simulink model "battery_model"  (R2021a)
settings: Solver=VariableStepAuto  StartTime=0.0  StopTime=10.0  RelTol=1e-3
libraries: fl_lib x5, nesl_utility x5, ee_lib x1
settings Model: Creator=shubh  LastModifiedBy=LENOVO

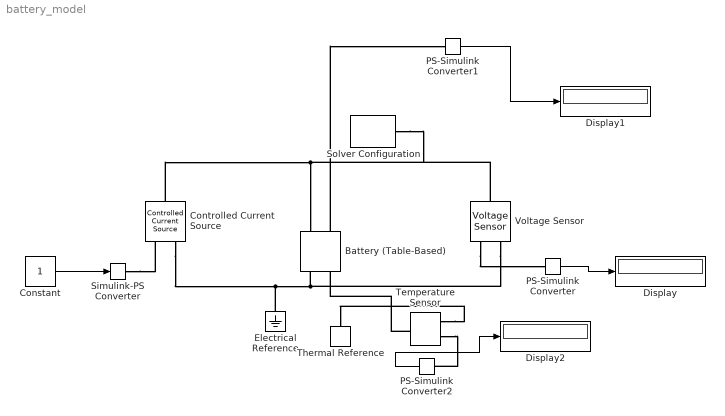
== system battery_model ==
  Battery (Table-Based) : ee_lib/Sources/Battery (Table-Based)  Tag={'toolbox/physmod/elec/library/m/ee_lib_parts';'Sources/Battery__Table_Based_/Panasonic/NCA103450.xml'}  SOC_vec=[0 0.01 0.02 0.03 0.04 0.05 0.06 0.07 0.08 0.09 0.1 0.11 0.12 0.13 0.14 0.15 0.16 0.17 0.18 0.19 0.2 0.21 0.22 0.23 0.24 0.25 0.26 0.27 0.28 0.29 0.3 0.31 0.32 0.33 0.34 0.35 0.36 0.37 0.38 0.39 0.4 0.41 0.42 0.43 0.44 0.45 0.46 0.47 0.48 0.49 0.5 0.51 0.52 0.53 0.54 0.55 0.56 0.57 0.58 0.59 0.6 0.61 0.62 0.63 0.64 0.65 0.66 0.67 0.68 0.69 0.7 0.71 0.72 0.73 0.74 0.75 0.76 0.77 0.78 0.79 0.8 0.81 0.82 0.83 0.84 0.85 0.86 0.87 0.88 0.89 0.9 0.91 0.92 0.93 0.94 0.95 0.96 0.97 0.98 0.99 1]  T_dependence=ee.enum.temperature_dependence.yes  prm_dir=ee.enum.battery.prm_dir.noCurrentDirectionality  T_vec=[-20 -10 0 25 40] degC  V0_mat=[3.05694324577171 3.05694324577171 3.05694324577171 3.05694324577171 3.05694324577171;3.11780933073521 3.11780933073521 3.11780933073521 3.11780933073521 3.11780933073521;3.16456091699536 3.16456091699536 3.16456091699536 3.16456091699536 3.16456091699536;3.20312763991407 3.20312763991407 3.20312763991407 3.20312763991407 3.20312763991407;3.23988086559703 3.23988086559703 3.23988086559703 3.23988086559703 3.23988086559703;3.27357083912107 3.27357083912107 3.27357083912107 3.27357083912107 3.27357083912107;3.29790581816648 3.29790581816648 3.29790581816648 3.29790581816648 3.29790581816648;3.31993534905873 3.31993534905873 3.31993534905873 3.31993534905873 3.31993534905873;3.34081960093889 3.34081960093889 3.34081960093889 3.34081960093889 3.34081960093889;3.35851365985912 3.35851365985912 3.35851365985912 3.35851365985912 3.35851365985912;3.37584043549754 3.37584043549754 3.37584043549754 3.37584043549754 3.37584043549754;3.39148360721865 3.39148360721865 3.39148360721865 3.39148360721865 3.39148360721865;3.40552818269083 3.40552818269083 3.40552818269083 3.40552818269083 3.40552818269083;3.41727372987041 3.41727372987041 3.41727372987041 3.41727372987041 3.41727372987041;3.42829270908039 3.42829270908039 3.42829270908039 3.42829270908039 3.42829270908039;3.43848498572673 3.43848498572673 3.43848498572673 3.43848498572673 3.43848498572673;3.44779771527731 3.44779771527731 3.44779771527731 3.44779771527731 3.44779771527731;3.45685827606495 3.45685827606495 3.45685827606495 3.45685827606495 3.45685827606495;3.46591883685259 3.46591883685259 3.46591883685259 3.46591883685259 3.46591883685259;3.47482240360815 3.47482240360815 3.47482240360815 3.47482240360815 3.47482240360815;3.48166780164756 3.48166780164756 3.48166780164756 3.48166780164756 3.48166780164756;3.48730800046594 3.48730800046594 3.48730800046594 3.48730800046594 3.48730800046594;3.49312425534464 3.49312425534464 3.49312425534464 3.49312425534464 3.49312425534464;3.49938346777656 3.49938346777656 3.49938346777656 3.49938346777656 3.49938346777656;3.50564268020849 3.50564268020849 3.50564268020849 3.50564268020849 3.50564268020849;3.51179877842532 3.51179877842532 3.51179877842532 3.51179877842532 3.51179877842532;3.5177347500538 3.5177347500538 3.5177347500538 3.5177347500538 3.5177347500538;3.52360520400279 3.52360520400279 3.52360520400279 3.52360520400279 3.52360520400279;3.5293131703325 3.5293131703325 3.5293131703325 3.5293131703325 3.5293131703325;3.53495846514988 3.53495846514988 3.53495846514988 3.53495846514988 3.53495846514988;3.54064002733928 3.54064002733928 3.54064002733928 3.54064002733928 3.54064002733928;3.5466862346196 3.5466862346196 3.5466862346196 3.5466862346196 3.5466862346196;3.55275206033938 3.55275206033938 3.55275206033938 3.55275206033938 3.55275206033938;3.55881788605916 3.55881788605916 3.55881788605916 3.55881788605916 3.55881788605916;3.56471104033438 3.56471104033438 3.56471104033438 3.56471104033438 3.56471104033438;3.57059107321653 3.57059107321653 3.57059107321653 3.57059107321653 3.57059107321653;3.57650036036778 3.57650036036778 3.57650036036778 3.57650036036778 3.57650036036778;3.58267113851687 3.58267113851687 3.58267113851687 3.58267113851687 3.58267113851687;3.58862363879637 3.58862363879637 3.58862363879637 3.58862363879637 3.58862363879637;3.59455112950322 3.59455112950322 3.59455112950322 3.59455112950322 3.59455112950322;3.60047862021008 3.60047862021008 3.60047862021008 3.60047862021008 3.60047862021008;3.60621921690956 3.60621921690956 3.60621921690956 3.60621921690956 3.60621921690956;3.61193277295345 3.61193277295345 3.61193277295345 3.61193277295345 3.61193277295345;3.61764632899735 3.61764632899735 3.61764632899735 3.61764632899735 3.61764632899735;3.62335988504124 3.62335988504124 3.62335988504124 3.62335988504124 3.62335988504124;3.62907344108513 3.62907344108513 3.62907344108513 3.62907344108513 3.62907344108513;3.63478699712903 3.63478699712903 3.63478699712903 3.63478699712903 3.63478699712903;3.64052178962629 ...(+4558 chars)] V  V0_vec=[3.05694324577171 3.11780933073521 3.16456091699536 3.20312763991407 3.23988086559703 3.27357083912107 3.29790581816648 3.31993534905873 3.34081960093889 3.35851365985912 3.37584043549754 3.39148360721865 3.40552818269083 3.41727372987041 3.42829270908039 3.43848498572673 3.44779771527731 3.45685827606495 3.46591883685259 3.47482240360815 3.48166780164756 3.48730800046594 3.49312425534464 3.49938346777656 3.50564268020849 3.51179877842532 3.5177347500538 3.52360520400279 3.5293131703325 3.53495846514988 3.54064002733928 3.5466862346196 3.55275206033938 3.55881788605916 3.56471104033438 3.57059107321653 3.57650036036778 3.58267113851687 3.58862363879637 3.59455112950322 3.60047862021008 3.60621921690956 3.61193277295345 3.61764632899735 3.62335988504124 3.62907344108513 3.63478699712903 3.64052178962629 3.64808511653063 3.65679215163517 3.66549918673971 3.6742776274848 3.68308819862471 3.69189876976462 3.70070934090453 3.70951991204444 3.71829251081983 3.72662762793713 3.73481883068441 3.74300361156379 3.75096334989971 3.75892308823563 3.76688282657154 3.77484256490746 3.78285738534165 3.79096087292362 3.79907208206368 3.80718329120375 3.81529450034382 3.82340570948388 3.83152467609174 3.83977969842631 3.84803472076089 3.85689864431254 3.8665947233018 3.87644566188505 3.88631890813263 3.89619215438021 3.90606540062778 3.91593864687536 3.92581189312294 3.93568513937051 3.94640464120662 3.95745251209717 3.96864585088705 3.98047153819836 3.9924662722967 4.00446100639504 4.01645574049338 4.02845047459172 4.03962340380677 4.05026614066205 4.06069004513023 4.07111394959842 4.08126368305597 4.09164730401325 4.10347838409614 4.11623674377326 4.12666159839296 4.13378671073504 4.05293761327992] V  R0_mat=[0.141685622669533 0.144330670296816 0.145951810032112 0.0876729363384268 0.146321047773631;0.160963346658006 0.160698886191678 0.150906802623426 0.0932229543109529 0.12440875553873;0.173825389417679 0.17065142085774 0.14944611398594 0.0950081088191402 0.108002561492024;0.182967039749425 0.176883563095875 0.144265032920527 0.0963551224210397 0.109029380824381;0.191284373155831 0.182291388408669 0.147971901771216 0.0982529232972309 0.109231883231397;0.198209319217276 0.188395970195294 0.152775341587345 0.100527086809133 0.108041998293454;0.202056790677236 0.190736653273694 0.153326511185911 0.100635443372933 0.102599843137946;0.205007765369114 0.192029405373389 0.152829749805771 0.100924551895045 0.105416708079588;0.207438158691858 0.19280157610395 0.151812407056497 0.101472051142568 0.108218448748171;0.208418464305548 0.192123659125456 0.152607874905011 0.101627556367249 0.109570101707698;0.209231822972955 0.19127879520068 0.153587839714389 0.101741529793572 0.110754807720943;0.210343575742801 0.191833133998348 0.153802530015898 0.101999894636474 0.111174239226319;0.210906938107855 0.191939665053811 0.153290585658805 0.101899166770183 0.110867036073093;0.210425287612639 0.191001183249004 0.151733628441442 0.101204214783437 0.109514820059597;0.209613378949417 0.18973244327619 0.149846413056072 0.101035811125123 0.107832345878095;0.208425696393633 0.188087929410814 0.147583423778142 0.100938308201256 0.105774097804031;0.206838219703417 0.186043621411006 0.144920640365778 0.100646635129898 0.1048982342853;0.205136120848225 0.183884691246222 0.144265334326882 0.100298317383989 0.104783849816211;0.204781000088455 0.18172576108144 0.144096514624598 0.0999499996380807 0.104669465347122;0.204845388629513 0.180789899114949 0.143856333998639 0.099556199105654 0.104483719954358;0.203974245935958 0.179205361561599 0.142680622138068 0.098627385343966 0.103362443326983;0.202555285414659 0.177073006180505 0.140957092449753 0.0976208329780398 0.101693348871863;0.201216350375327 0.175020676281377 0.139313588243404 0.0967773657175446 0.10010427989871;0.200078759678369 0.173169690724624 0.137871428379431 0.0963442210505122 0.0987165552679319;0.198941168981411 0.171318705167871 0.136429268515457 0.0959110763834798 0.0973288306371532;0.197756708186686 0.169420849513351 0.134940238553716 0.0954547691681331 0.0958942359086076;0.196472189851799 0.167422936318669 0.133351151051812 0.0949490149125893 0.0943595836398997;0.195157890753505 0.16539524236058 0.131732282786502 0.0944242795111379 0.0927951506077853;0.194078713655907 0.163293690393728 0.130039556512429 0.0939040760935132 0.0911568595669077;0.193117191689189 0.16189590605745 0.129087926592782 0.0933892475911817 0.0899127547919209;0.192172154891564 0.16081228938684 0.128373215654712 0.0929080144571439 0.0892588989120233;0.191392865862544 0.159894420484837 0.127824252485248 0.0927344186869696 0.0887707908007316;0.190622494306004 0.158985469055313 0.127284206788263 0.0925652298072645 0.0882916001619189;0.189852122749463 0.158076517625787 0.126744161091277 0.092396040927559 0.0878124095231052;0.189003264172671 0.157089079176012 0.126125628374041 0.0921768273536275 0.0872547318640409;0.188148441326298 0.156095676456655 0.125501131387224 0.0919538123771066 0.0866910899353958;0.187306915874968 0.155115571132341 0.12488993179545 0.091728288458123 0.0861407454017938;0.186584249968117 0.154254325352506 0.124397591748154 0.0914803382099938 0.0857092604126705;0.185973999931887 0.153293862359217 0.123806034487405 0.0911833561994023 0.0851785582100926;0.185407583884335 0.152322031378363 0.123203109239091 0.0908807562879789 0.0846364880199505;0.184841167836782 0.151350200397509 0.122600183990775 0.0905781563765555 0.0840944178298075;0.184189799967698 0.150293417595122 0.121806624470283 0.0901024318999258 0.0834673958181323;0.183526140891528 0.149405957488493 0.12081808813039 0.0896016589917948 0.0828280825993722;0.182862481815358 0.148580232764828 0.119829551790498 0.0891008860836628 0.0821887693806117 ...(+5198 chars)] Ohm  R0_vec=[0.0876729363384268 0.0932229543109529 0.0950081088191402 0.0963551224210397 0.0982529232972309 0.100527086809133 0.100635443372933 0.100924551895045 0.101472051142568 0.101627556367249 0.101741529793572 0.101999894636474 0.101899166770183 0.101204214783437 0.101035811125123 0.100938308201256 0.100646635129898 0.100298317383989 0.0999499996380807 0.099556199105654 0.098627385343966 0.0976208329780398 0.0967773657175446 0.0963442210505122 0.0959110763834798 0.0954547691681331 0.0949490149125893 0.0944242795111379 0.0939040760935132 0.0933892475911817 0.0929080144571439 0.0927344186869696 0.0925652298072645 0.092396040927559 0.0921768273536275 0.0919538123771066 0.091728288458123 0.0914803382099938 0.0911833561994023 0.0908807562879789 0.0905781563765555 0.0901024318999258 0.0896016589917948 0.0891008860836628 0.0886001131755307 0.0880993402673991 0.087598567359268 0.0871039468701925 0.0871146616224242 0.0872948764839462 0.0874750913454692 0.087721451026969 0.0879975738919554 0.0882736967569409 0.0885498196219272 0.0888259424869137 0.0890668906066512 0.0889393184390105 0.0888240888416965 0.0887072256611772 0.0885368621772216 0.0883664986932668 0.0881961352093101 0.0880257717253553 0.0879064321583712 0.0878659140766787 0.0878247337687346 0.0877835534607895 0.0877423731528449 0.0877011928449002 0.087661755097109 0.087652879550087 0.0876440040030652 0.0879694121511781 0.088545618141283 0.0891085428626062 0.0896695544051722 0.0902305659477382 0.0907915774903036 0.091352589032869 0.0919136005754355 0.092474612118 0.0932257180713086 0.0940612343386086 0.094932150401911 0.0962822749828668 0.0977889918051445 0.0992957086274227 0.100802425449702 0.10230914227198 0.10363125704595 0.104982100658977 0.106351712058201 0.107721323457427 0.108820835674904 0.109987805318691 0.111479917736467 0.112737722386497 0.109961816871439 0.104129278053125 0.01680404166307] Ohm  R0_dis_mat=[0.03 0.015 0.002;0.04 0.017 0.008;0.039 0.012 0.006;0.027 0.013 0.021] % Parameter not set Ohm  R0_dis_vec=[0.015 0.017 0.012 0.013] % Parameter not set Ohm  R0_ch_mat=[0.03 0.015 0.002;0.04 0.017 0.008;0.039 0.012 0.006;0.027 0.013 0.021] % Parameter not set Ohm  R0_ch_vec=[0.015 0.017 0.012 0.013] % Parameter not set Ohm  AH_vec=[1.55869476118114 1.8607446859296 2.01137468341514 2.193305986659 2.31762046623156] hr*A  AH=2.193305986659 hr*A  prm_leak=ee.enum.battery.prm_leak.disabled  Rleak_vec=[8000 7000 6000] % Parameter not set Ohm  Rleak=7000 % Parameter not set Ohm  extrapolation_option=ee.enum.extrapolation.nearest  prm_dyn=ee.enum.battery.prm_dyn.off  R1_mat=[0.089 0.076 0.01;0.042 0.022 0.099;0.019 0.007 0.002;0.051 0.043 0.029] % Parameter not set Ohm  R1_vec=[0.076 0.022 0.007 0.043] % Parameter not set Ohm  tau1_mat=[44 148 235;93 110 1000;19 27 133;0.5 22 3] % Parameter not set s  tau1_vec=[148 110 27 22] % Parameter not set s  R2_mat=[0.014 0.382 0.407;0.028 0.006 0.007;0.014 0.007 0.006;0.333 0.956 0.912] % Parameter not set Ohm  R2_vec=[0.382 0.006 0.007 0.956] % Parameter not set Ohm  tau2_mat=[1 44 5644;11 24 506;2 14 330;3310 13419 30216] % Parameter not set s  tau2_vec=[44 24 14 13419] % Parameter not set s  R3_mat=[0.014 0.382 0.407;0.028 0.006 0.007;0.014 0.007 0.006;0.333 0.956 0.912] % Parameter not set Ohm  R3_vec=[0.382 0.006 0.007 0.956] % Parameter not set Ohm  tau3_mat=[1 44 5644;11 24 506;2 14 330;3310 13419 30216] % Parameter not set s  tau3_vec=[44 24 14 13419] % Parameter not set s  R4_mat=[0.014 0.382 0.407;0.028 0.006 0.007;0.014 0.007 0.006;0.333 0.956 0.912] % Parameter not set Ohm  R4_vec=[0.382 0.006 0.007 0.956] % Parameter not set Ohm  tau4_mat=[1 44 5644;11 24 506;2 14 330;3310 13419 30216] % Parameter not set s  tau4_vec=[44 24 14 13419] % Parameter not set s  R5_mat=[0.014 0.382 0.407;0.028 0.006 0.007;0.014 0.007 0.006;0.333 0.956 0.912] % Parameter not set Ohm  R5_vec=[0.382 0.006 0.007 0.956] % Parameter not set Ohm  tau5_mat=[1 44 5644;11 24 506;2 14 330;3310 13419 30216] % Parameter not set s  tau5_vec=[44 24 14 13419] % Parameter not set s  prm_fade=ee.enum.battery.prm_fade.tableN  N0=100 % Parameter not set  dV0=0 % Parameter not set  dR0=0 % Parameter not set  dAH=0 % Parameter not set  dRleak=0 % Parameter not set  dR1=0 % Parameter not set  dR2=0 % Parameter not set  dR3=0 % Parameter not set  dR4=0 % Parameter not set  dR5=0 % Parameter not set  N0vec=[1 6 11 16 21 26 31 36 41 46 51 56 61 66 71 76 81 86 91 96 101 106 111 116 121 126 131 136 141 146 151 156 161 166 171 176 181 186 191 196 201 206 211 216 221 226 231 236 241 246 251 256 261 266 271 276 281 286 291 296 301 306 311 316 321 326 331 336 341 346 351 356 361 366 371 376 381 386 391 396 401 406 411 416 421 426 431 436 441 446 451 456 461 466 471 476 481 486 491 496]  Tfadevec=[298.15 323.15] % Parameter not set K  dV0vec=[0 1.10576459758607 1.97572945152668 1.87828003984863 1.76314184449295 1.62056220493866 1.56247815839591 1.52003609404217 1.47744416806089 1.43485224207961 1.39226031609831 1.34966839011701 1.30707646413573 1.26448453815445 1.22371856658483 1.18422222850361 1.14135385798404 1.09050719258034 1.0396605271766 0.988813861772903 0.940063540749295 0.895437648878542 0.85081175700779 0.806185865137015 0.761559973266241 0.71693408139551 0.672907210282603 0.629286501316299 0.585665792349996 0.542045083383692 0.506686498509871 0.471972266399757 0.436955084942783 0.4013031300697 0.365651175196617 0.329999220323534 0.294347265450451 0.258695310577368 0.223043355704285 0.187391400831202 0.151739445958163 0.11608749108508 0.0804355362120185 0.0447835813389573 0.00913162646587428 -0.0168261289375092 -0.035088995065174 -0.0533518611928607 -0.0717343945200007 -0.0903806588841135 -0.109026923248226 -0.127673187612339 -0.146319451976452 -0.164965716340565 -0.183611980704678 -0.202258245068791 -0.220904509432904 -0.239550773797016 -0.258197038161129 -0.279035070103965 -0.312374631634333 -0.346571377380647 -0.381571825677453 -0.41657227397426 -0.451572722271067 -0.486573170567873 -0.521573618864702 -0.556574067161487 -0.591574515458315 -0.628222003502564 -0.665796847356149 -0.703371691209755 -0.740946535063362 -0.776248754132794 -0.803500841123046 -0.830752928113297 -0.858005015103527 -0.885257102093779 -0.912509189084031 -0.939761276074282 -0.967013363064534 -0.994265450054808 -1.02151753704506 -1.04876962403531 -1.07602171102556 -1.10327379801584 -1.1303726689468 -1.14505002807567 -1.15972738720453 -1.17440474633339 -1.18908210546226 -1.20375946459112 -1.21843682371996 -1.23311418284882 -1.24779154197769 -1.26246890110655 -1.27714626023541 -1.29182361936425 -1.30650097849312 -1.32117833762196]  dR0vec=[0;0;0;0;0;0;0;0;0;0;0;0;0;0;0;0;0;0;0;0;0;0;0;0;0;0;0;0;0;0;0;0;0;0;0;0;0;0;0;0;0;0;0;0;0;0;0;0;0;0;0;0;0;0;0;0;0;0;0;0;0;0;0;0;0;0;0;0;0;0;0;0;0;0;0;0;0;0;0;0;0;0;0;0;0;0;0;0;0;0;0;0;0;0;0;0;0;0;0;0] % Parameter not set  dAHvec=[0 -0.554316012182733 -1.1086320243655 -1.66294803654826 -2.21726404873103 -2.77158006091378 -2.99739713515845 -3.13269855571741 -3.26799997627637 -3.40330139683531 -3.53860281739426 -3.67390423795322 -3.80920565851216 -3.94450707907112 -4.07980849963007 -4.21510992018901 -4.36196281111826 -4.53614670750021 -4.71033060388216 -4.88451450026413 -5.05869839664608 -5.23288229302803 -5.40706618940998 -5.58125008579193 -5.7554339821739 -5.92961787855585 -6.1038017749378 -6.27798567131975 -6.4521695677017 -6.62635346408365 -6.76754548571347 -6.90616451213779 -7.04478353856213 -7.18340256498647 -7.32202159141079 -7.46064061783513 -7.59925964425945 -7.73787867068379 -7.87649769710813 -8.01511672353245 -8.15373574995677 -8.29235477638112 -8.43097380280546 -8.56959282922977 -8.70821185565412 -8.80913868547283 -8.88014687370122 -8.95115506192963 -9.02216325015801 -9.0931714383864 -9.16417962661481 -9.23518781484319 -9.30619600307157 -9.37720419129998 -9.44821237952837 -9.51922056775675 -9.59022875598516 -9.66123694421355 -9.73224513244195 -9.81159994934316 -9.93856274544924 -10.0655255415553 -10.1924883376614 -10.3194511337675 -10.4464139298736 -10.5733767259797 -10.7003395220858 -10.8273023181919 -10.954265114298 -11.0812279104041 -11.2081907065101 -11.3351535026162 -11.4621162987223 -11.5814000530147 -11.6734829683154 -11.7655658836161 -11.8576487989168 -11.9497317142175 -12.0418146295181 -12.1338975448188 -12.2259804601195 -12.3180633754202 -12.4101462907209 -12.5022292060216 -12.5943121213223 -12.686395036623 -12.7779602454664 -12.8275540258614 -12.8771478062564 -12.9267415866515 -12.9763353670465 -13.0259291474415 -13.0755229278365 -13.1251167082315 -13.1747104886265 -13.2243042690216 -13.2738980494166 -13.3234918298116 -13.3730856102066 -13.4226793906016]  dRleakvec=[0 0 0] % Parameter not set  dR1vec=[0 0 0] % Parameter not set  dR2vec=[0 0 0] % Parameter not set  dR3vec=[0 0 0] % Parameter not set  dR4vec=[0 0 0] % Parameter not set  dR5vec=[0 0 0] % Parameter not set  dV0mat=[0 0;0 0;0 0] % Parameter not set  dR0mat=[0 0;0 0;0 0] % Parameter not set  dAHmat=[0 0;0 0;0 0] % Parameter not set  dRleakmat=[0 0;0 0;0 0] % Parameter not set  dR1mat=[0 0;0 0;0 0] % Parameter not set  dR2mat=[0 0;0 0;0 0] % Parameter not set  dR3mat=[0 0;0 0;0 0] % Parameter not set  dR4mat=[0 0;0 0;0 0] % Parameter not set  dR5mat=[0 0;0 0;0 0] % Parameter not set  prm_age=ee.enum.battery.prm_age.disabled  prm_age_OCV=ee.enum.battery.prm_age_OCV.SOC  OCV_age=0.9 % Parameter not set  SOC_age=0.6 % Parameter not set  storage_dt_age_vec=0 % Parameter not set d  storage_T_age_vec=273 % Parameter not set K  OCV_scaling_age=2213400 % Parameter not set  OCV_offset_age=1632000 % Parameter not set  temp_exp_age=0.515833569 % Parameter not set V  t_exp_age=0.75 % Parameter not set  T_age_vec=[273.15 298.15 323.15] % Parameter not set K  dt_age_vec=[90 180 270 360] % Parameter not set d  dR0_age_vec=[0 0 0] % Parameter not set  t_meas_dR0_age=100 % Parameter not set d  dR0_age_mat=[0 0 0;0 0 0;0 0 0;0 0 0] % Parameter not set  temperature=298.15 K  i_specify=off  i_priority=None  i=0 A  i_nominal_specify=off  i_nominal_unit=A  i_nominal_value=1  v_specify=off  v_priority=None  v=0 V  v_nominal_specify=off  v_nominal_unit=V  v_nominal_value=1  stateOfCharge_specify=off  stateOfCharge_priority=High  stateOfCharge=1  stateOfCharge_nominal_specify=off  stateOfCharge_nominal_unit=1  stateOfCharge_nominal_value=1  num_cycles_specify=off  num_cycles_priority=High  num_cycles=0  num_cycles_nominal_specify=off  num_cycles_nominal_unit=1  num_cycles_nominal_value=1  thermal_mass=30000 % Parameter not set J/K  temperature_specify=off  temperature_priority=High  temperature_nominal_specify=off  temperature_nominal_unit=K  temperature_nominal_value=1
      settings: AttributesFormatString=Panasonic:NCA103450  SourceProductBaseCode=PS  InternalSimscapePortConfiguration="{\"Bottom\":[],\"Left\":[{\"id\":\"p\",\"label\":\"+\",\"type\":\"foundation.electrical.electrical\"},{\"id\":\"soc\",\"label\":\"SOC\",\"type\":\"output\"}],\"Right\":[{\"id\":\"n\",\"label\":\"-\",\"type\":\"foundation.electrical.electrical\"},{\"id\":\"H\",\"label\":\"H\",\"type\":\"foundation.thermal.thermal\"}],\"Top\":[]}"
  Constant : Constant
  Controlled Current Source : fl_lib/Electrical/Electrical Sources/Controlled Current Source
  Display : Display
  Display1 : Display
  Display2 : Display
  Electrical Reference : fl_lib/Electrical/Electrical Elements/Electrical Reference
  PS-Simulink Converter : nesl_utility/PS-Simulink Converter  PhysicalDomain=network_engine_domain  SubClassName=ps_output  LeftPortType=input  RightPortType=output  PseudoPeriodic=off  Frequencies=[]  Unit=inherit  AffineConversion=off
      settings: SourceProductBaseCode=PW,SS
  PS-Simulink Converter1 : nesl_utility/PS-Simulink Converter  PhysicalDomain=network_engine_domain  SubClassName=ps_output  LeftPortType=input  RightPortType=output  PseudoPeriodic=off  Frequencies=[]  Unit=inherit  AffineConversion=off
      settings: SourceProductBaseCode=PW,SS
  PS-Simulink Converter2 : nesl_utility/PS-Simulink Converter  PhysicalDomain=network_engine_domain  SubClassName=ps_output  LeftPortType=input  RightPortType=output  PseudoPeriodic=off  Frequencies=[]  Unit=inherit  AffineConversion=off
      settings: SourceProductBaseCode=PW,SS
  Simulink-PS Converter : nesl_utility/Simulink-PS Converter  PhysicalDomain=network_engine_domain  SubClassName=ps_input  LeftPortType=input  RightPortType=output  PseudoPeriodic=off  Frequencies=[]  NoiseDistribution=none  NoiseParameters=[]  Unit=1  AffineConversion=off  FilteringAndDerivatives=provide  SimscapeFilterOrder=1  InputFilterTimeConstant=0.001  UdotUserProvided=0
      settings: SourceProductBaseCode=PW,SS
  Solver Configuration : nesl_utility/Solver Configuration  PhysicalDomain=network_engine_domain  SubClassName=solver  LeftPortType=input  RightPortType=generic  Tones=[]  Harmonics=[]  SimulateNoise=off  Profile=off  UseLocalSampling=off  EnableSwitchedLinearOptims=on  FrequencyDomain=off  UseCCode=off  RelTol=0.001  AbsTol=1e-06  MinStep=1e-09  ToWorkspace=off  RevertToSquareIcSolve=off  NumHomotopyIterations=100  PhasorMode=off  PhasorModeNumHarmonics=1  DoDC=off  ResidualTolerance=1e-09  UseLocalSolver=off  LocalSolverChoice=NE_BACKWARD_EULER_ADVANCER  LocalSolverSampleTime=0.001  DoFixedCost=off  MaxNonlinIter=3  MaxModeIter=2  ComputeImpulses=off  ImpulseIterations=2  LinearAlgebra=auto  EquationFormulation=NE_TIME_EF  DelaysMemoryBudget=1024  AutomaticFiltering=on  FilteringTimeConstant=0.001  PartitionStorageMethod=AS_NEEDED  PartitionMemoryBudget=1024  PartitionMethod=ROBUST
      settings: SourceProductBaseCode=PW,SS
  Temperature Sensor : fl_lib/Thermal/Thermal Sensors/Temperature Sensor
  Thermal Reference : fl_lib/Thermal/Thermal Elements/Thermal Reference
  Voltage Sensor : fl_lib/Electrical/Electrical Sensors/Voltage Sensor
  wires:
  Constant/1 -> Simulink-PS Converter/1
  PS-Simulink Converter/1 -> Display/1
  PS-Simulink Converter1/1 -> Display1/1
  PS-Simulink Converter2/1 -> Display2/1
  connections:
  Simulink-PS Converter/RConn1 -- Controlled Current Source/RConn1
  Controlled Current Source/RConn2 -- Voltage Sensor/RConn2 -- Battery (Table-Based)/RConn1 -- Electrical Reference/LConn1
  Controlled Current Source/LConn1 -- Solver Configuration/RConn1 -- Voltage Sensor/LConn1 -- Battery (Table-Based)/LConn1
  Voltage Sensor/RConn1 -- PS-Simulink Converter/LConn1
  Battery (Table-Based)/LConn2 -- PS-Simulink Converter1/LConn1
  Temperature Sensor/RConn1 -- Thermal Reference/LConn1
  Temperature Sensor/LConn1 -- Battery (Table-Based)/RConn2
  Temperature Sensor/RConn2 -- PS-Simulink Converter2/LConn1
